simulink model "pendulo"  (R2021a)
settings: Solver=VariableStepAuto  StartTime=0.0  StopTime=10.0  RelTol=1e-3
values from neighbouring files (symbols this model uses):
  A = eval(A)    [E2_puntos_equilibrio.m]    (also in E4_nyquist2.m = 0:0.01:10)
  B = eval(B)    [E2_puntos_equilibrio.m]
  C = [1 0]    [E2_puntos_equilibrio.m]
  D = 0    [E2_puntos_equilibrio.m]
  x0 = 0.9    [E1_puntos_equilibrio.m]    (also in E2_puntos_equilibrio.m = [x10;0])
  x1 = 0    [E2_puntos_equilibrio.m]
  x10 = 0.3    [E2_puntos_equilibrio.m]
settings Model: Creator=OSCAR  LastModifiedBy=OSCAR

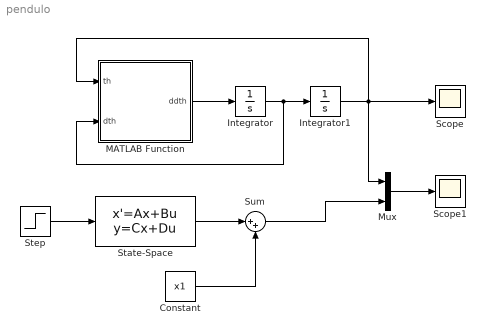
== system pendulo ==
  Constant : Constant  Value=x1
  Integrator : Integrator
  Integrator1 : Integrator  InitialCondition=x10
  MATLAB Function : MATLAB Function  TreatAsAtomicUnit=on
  Mux : Mux  Inputs=2
  Scope : Scope
  Scope1 : Scope
  State-Space : StateSpace  A=A  B=B  C=C  D=D  InitialCondition=x0
  Step : Step  After=0  SampleTime=0
  Sum : Sum  Inputs=|++
  wires:
  MATLAB Function/1(ddth) -> Integrator/1
  Integrator/1 -> MATLAB Function/2(dth), Integrator1/1
  Integrator1/1 -> Mux/1, MATLAB Function/1(th), Scope/1
  Step/1 -> State-Space/1
  State-Space/1 -> Sum/1
  Constant/1 -> Sum/2
  Mux/1 -> Scope1/1
  Sum/1 -> Mux/2

== matlab function pendulo/MATLAB Function ==
  data: th input; ddth output; dth input
function ddth = pendulo(th,dth)

m=0.2;
g=9.81;
l=0.45;
B=0.15;
J=m*l^2;

ddth=-B/J*dth-m*g*l/J*sin(th);
